simulink model "progetto"  (R2021b)
settings: Solver=VariableStepAuto  StartTime=0.0  StopTime=5  RelTol=1e-3
values from neighbouring files (symbols this model uses):
  DD = 3*10^(-5)    (= 3e-05)    [progetto.m]
  denG = deG{1}    [progetto.m]
  denR = deR{1}    [progetto.m]
  NN = 2*10^(-4)    (= 0.0002)    [progetto.m]
  numG = nuG{1}    [progetto.m]
  numR = nuR{1}    [progetto.m]
  ue = b2*sqrt((K*M)/x03)    [progetto.m]
  WW = 8*10^(-5)    (= 8e-05)    [progetto.m]
  x = [1,2,3,4]    [progetto.m]
  x01 = sqrt((K*M)/(x3^3))    [progetto.m]
  x02 = 0    [progetto.m]
  x03 = 3*10^7    (= 30000000)    [progetto.m]
  ye = x01    [progetto.m]
settings Model: Creator=Gianmiriano  LastModifiedBy=Gianmiriano

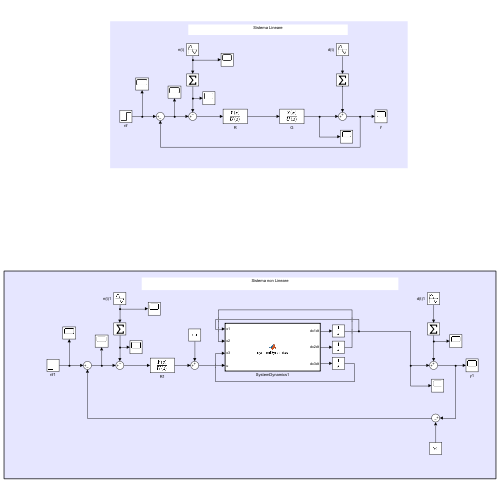
[thumbnail: Simulink's stored preview of the top-level diagram]
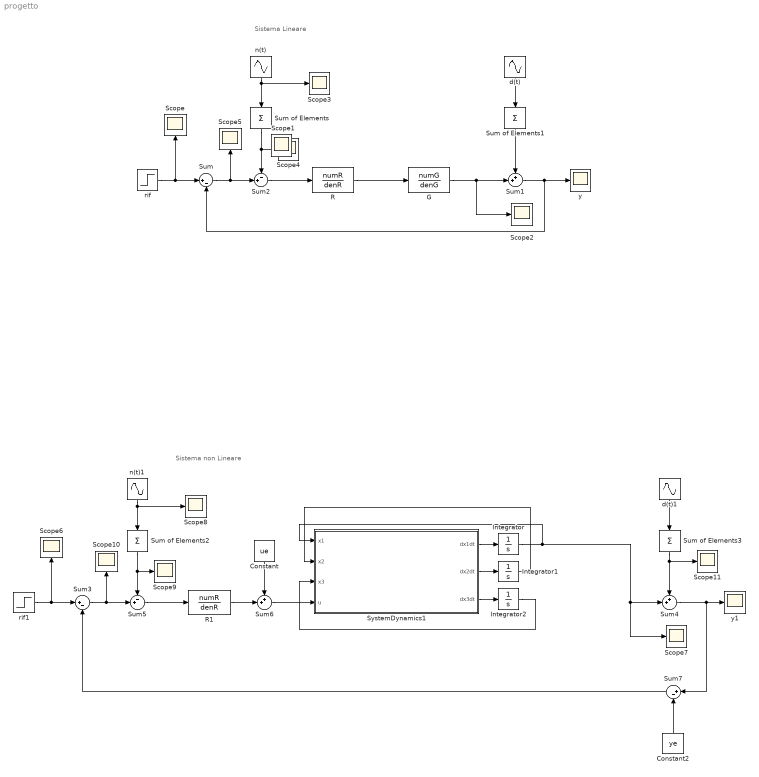
== system progetto ==
  note: Sistema Lineare
  note: Sistema non Lineare
  Constant : Constant  Value=ue
  Constant2 : Constant  Value=ye
  G : TransferFcn  Numerator=numG  Denominator=denG
  Integrator : Integrator  InitialCondition=x01
  Integrator1 : Integrator  InitialCondition=x02
  Integrator2 : Integrator  InitialCondition=x03
  R : TransferFcn  Numerator=numR  Denominator=denR
  R1 : TransferFcn  Numerator=numR  Denominator=denR
  Scope{,1..11} (12 alike) : Scope
  Sum : Sum  Inputs=|+-
  Sum of Elements{,1..3} (4 alike) : Sum  Inputs=+  CollapseDim=4
  Sum1 : Sum  Inputs=++|
  Sum2 : Sum  Inputs=-+|
  Sum3 : Sum  Inputs=|+-
  Sum4 : Sum  Inputs=++|
  Sum5 : Sum  Inputs=-+|
  Sum6 : Sum  Inputs=++|
  Sum7 : Sum  Inputs=|+-
  SystemDynamics1 : MATLAB Function  TreatAsAtomicUnit=on
  d(t) : Sin  Amplitude=DD  Frequency=0.02*x  SampleTime=0
  d(t)1 : Sin  Amplitude=DD  Frequency=0.02*x  SampleTime=0
  n(t) : Sin  Amplitude=NN  Frequency=5*10^4*x  SampleTime=0
  n(t)1 : Sin  Amplitude=NN  Frequency=5*10^4*x  SampleTime=0
  rif : Step  Time=0  After=WW  SampleTime=0
  rif1 : Step  Time=0  After=WW  SampleTime=0
  y : Scope
  y1 : Scope
  wires:
  rif/1 -> Scope/1, Sum/1
  G/1 -> Scope2/1, Sum1/2
  Sum1/1 -> y/1, Sum/2
  n(t)/1 -> Sum of Elements/1, Scope3/1
  Sum of Elements/1 -> Sum2/1, Scope4/1
  d(t)/1 -> Sum of Elements1/1
  Sum of Elements1/1 -> Sum1/1
  Sum/1 -> Scope5/1, Sum2/2
  Sum2/1 -> R/1
  R/1 -> G/1
  Sum5/1 -> R1/1
  d(t)1/1 -> Sum of Elements3/1
  Sum of Elements3/1 -> Sum4/1, Scope11/1
  Sum3/1 -> Scope10/1, Sum5/2
  Sum4/1 -> Sum7/1, y1/1
  Sum of Elements2/1 -> Sum5/1, Scope9/1
  n(t)1/1 -> Sum of Elements2/1, Scope8/1
  rif1/1 -> Scope6/1, Sum3/1
  Integrator/1 -> SystemDynamics1/1(x1), Scope7/1, Sum4/2
  SystemDynamics1/1(dx1dt) -> Integrator/1
  SystemDynamics1/2(dx2dt) -> Integrator1/1
  SystemDynamics1/3(dx3dt) -> Integrator2/1
  Integrator1/1 -> SystemDynamics1/2(x2)
  Integrator2/1 -> SystemDynamics1/3(x3)
  R1/1 -> Sum6/2
  Sum6/1 -> SystemDynamics1/4(u)
  Constant/1 -> Sum6/1
  Constant2/1 -> Sum7/2
  Sum7/1 -> Sum3/2

== matlab function progetto/SystemDynamics1 ==
  data: x1 input; x2 input; x3 input; u input; dx1dt output; dx2dt output; dx3dt output
function [dx1dt, dx2dt, dx3dt] = systemDynamics(x1, x2, x3, u)
% sistema non linearizzato
b1=0.3;
b2=0.1;
m=1;
k=1.5;
K_G=6.67*10^(-11);
M=5.98*10^(24);

dx1dt=-(2*x1*x2)/x3-(b2*x1)/m+u/(m*x3);
dx2dt=(-b1*x2+m*(k-1)*(((K_G*M)/x3^2)-x3*(x1^2)))*1/m;
dx3dt=x2;
